simulink model "SVPWM"  (R2021a)
settings: Solver=VariableStepAuto  StartTime=0.0  StopTime=10.0  RelTol=1e-3
libraries: spsIGBTDiodeLib x6, spsSeriesRLCBranchLib x3, spsVoltageMeasurementLib x3, spsGroundLib x2, spsDCVoltageSourceLib x1, spsabctodq0Lib x1, spspowerguiLib x1
settings Model: Creator=User  LastModifiedBy=User

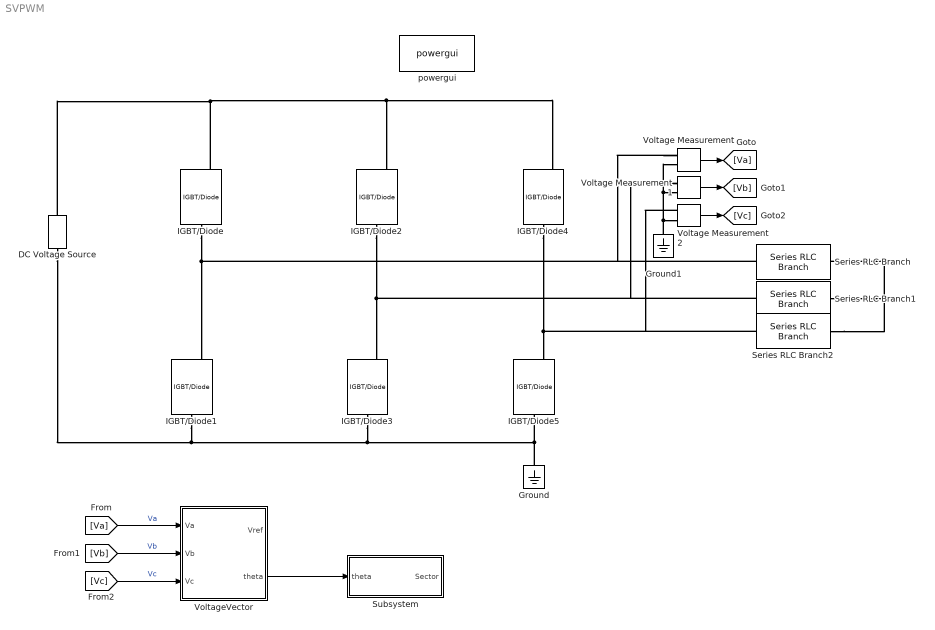
== system SVPWM ==
  DC Voltage Source : spsDCVoltageSourceLib/DC Voltage Source  Amplitude=100  Measurements=None
  Ground : spsGroundLib/Ground  LConnTagsString=a
  Ground1 : spsGroundLib/Ground  LConnTagsString=a
  IGBT/Diode{,1..5} (6 alike) : spsIGBTDiodeLib/IGBT//Diode  Ron=1e-3  Rs=1e5  Cs=inf  Measurements=off
  Series RLC Branch : spsSeriesRLCBranchLib/Series RLC Branch  LConnTagsString=__new0  RConnTagsString=__new0  BranchType=L  Resistance=1  Inductance=1e-3  SetiL0=off  InitialCurrent=0  Capacitance=1e-6  Setx0=off  InitialVoltage=0  Measurements=None
  Series RLC Branch1 : spsSeriesRLCBranchLib/Series RLC Branch  LConnTagsString=__new0  RConnTagsString=__new0  BranchType=L  Resistance=1  Inductance=1e-3  SetiL0=off  InitialCurrent=0  Capacitance=1e-6  Setx0=off  InitialVoltage=0  Measurements=None
  Series RLC Branch2 : spsSeriesRLCBranchLib/Series RLC Branch  LConnTagsString=__new0  RConnTagsString=__new0  BranchType=L  Resistance=1  Inductance=1e-3  SetiL0=off  InitialCurrent=0  Capacitance=1e-6  Setx0=off  InitialVoltage=0  Measurements=None
  Subsystem : Subsystem
  Voltage Measurement : spsVoltageMeasurementLib/Voltage Measurement  PhasorSimulation=off  OutputType=Complex  PSBequivalent=0
  Voltage Measurement1 : spsVoltageMeasurementLib/Voltage Measurement  PhasorSimulation=off  OutputType=Complex  PSBequivalent=0
  Voltage Measurement2 : spsVoltageMeasurementLib/Voltage Measurement  PhasorSimulation=off  OutputType=Complex  PSBequivalent=0
  VoltageVector : Subsystem
  powergui : spspowerguiLib/powergui  Priority=1  SimulationMode=Continuous  SampleTime=50e-6  frequency=60  Iterations=50  frequencyindice=60  Pbase=100e6  ErrMax=1e-4  UnitsV=kV  UnitsW=MW  buscounter=0  FunctionMessages=off  echomessages=off  EnableUseOfTLC=off  CurrentSourceSwitches=off  DisableSnubberDevices=off  DisableRonSwitches=off  DisableVfSwitches=off  DisplayEquations=off  AutomaticDiscreteSolvers=off  SolverType=Tustin/Backward Euler (TBE)  Interpol=off  ExternalGateDelay=off  methode=off  Ts=100  x0status=blocks  SPID=on  SwTol=0  HookPort=off  NonlinearTolerance=1e-4  nMaxIteration=100  ContinueOnMaxIteration=off  RestoreLinks=warning  ResistiveCurrentMeasurement=off  Frange=[0:2:500]  Ylog=off  Xlog=on  ShowGrid=off  save=off  variable=ZData  structure=0  ZoomFFT=off  StartTime=0.0  cycles=1  DisplayStyle=1  fundamental=60  FreqAxis=off  MaxFrequency=1000  frequencyindicesteady=1  RmsSteady=1  display=off
  wires:
  Voltage Measurement/1 -> [Va]
  Voltage Measurement1/1 -> [Vb]
  Voltage Measurement2/1 -> [Vc]
  [Va] -> VoltageVector/1(Va)  "Va"
  [Vb] -> VoltageVector/2(Vb)  "Vb"
  [Vc] -> VoltageVector/3(Vc)  "Vc"
  VoltageVector/2(theta) -> Subsystem/1(theta)
  connections:
  IGBT/Diode/LConn1 -- DC Voltage Source/RConn1 -- IGBT/Diode2/LConn1 -- IGBT/Diode4/LConn1
  IGBT/Diode2/RConn1 -- Voltage Measurement1/LConn1 -- Series RLC Branch1/LConn1 -- IGBT/Diode3/LConn1
  IGBT/Diode/RConn1 -- Voltage Measurement/LConn1 -- Series RLC Branch/LConn1 -- IGBT/Diode1/LConn1
  IGBT/Diode4/RConn1 -- Voltage Measurement2/LConn1 -- Series RLC Branch2/LConn1 -- IGBT/Diode5/LConn1
  IGBT/Diode1/RConn1 -- DC Voltage Source/LConn1 -- IGBT/Diode3/RConn1 -- Ground/LConn1 -- IGBT/Diode5/RConn1
  Series RLC Branch2/RConn1 -- Series RLC Branch1/RConn1 -- Series RLC Branch/RConn1
  Ground1/LConn1 -- Voltage Measurement1/LConn2 -- Voltage Measurement/LConn2 -- Voltage Measurement2/LConn2

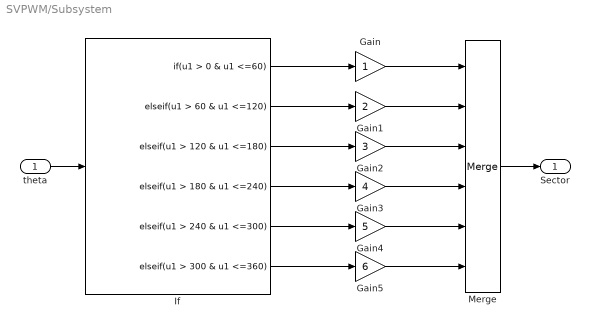
== system SVPWM/Subsystem ==
  theta : Inport
  Gain : Gain
  Gain1 : Gain  Gain=2
  Gain2 : Gain  Gain=3
  Gain3 : Gain  Gain=4
  Gain4 : Gain  Gain=5
  Gain5 : Gain  Gain=6
  If : If  IfExpression=u1 > 0 & u1 <=60  ElseIfExpressions=u1 > 60 & u1 <=120, u1 > 120 & u1 <=180, u1 > 180 & u1 <=240, u1 > 240 & u1 <=300, u1 > 300 & u1 <=360  ShowElse=off
  Merge : Merge  Inputs=6
  Sector : Outport
  wires:
  theta/1 -> If/1
  If/1 -> Gain/1
  If/2 -> Gain1/1
  If/3 -> Gain2/1
  If/4 -> Gain3/1
  If/5 -> Gain4/1
  If/6 -> Gain5/1
  Gain/1 -> Merge/1
  Gain1/1 -> Merge/2
  Gain2/1 -> Merge/3
  Gain3/1 -> Merge/4
  Gain4/1 -> Merge/5
  Gain5/1 -> Merge/6
  Merge/1 -> Sector/1

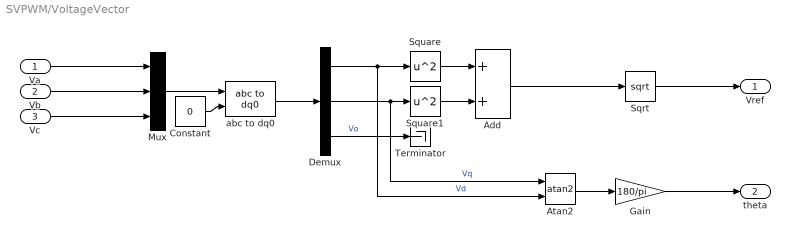
== system SVPWM/VoltageVector ==
  Va : Inport
  Vb : Inport  Port=2
  Vc : Inport  Port=3
  Add : Sum
  Atan2 : Trigonometry  Operator=atan2
  Constant : Constant  Value=0
  Demux : Demux  Outputs=3
  Gain : Gain  Gain=180/pi
  Mux : Mux  Inputs=3
      settings: DisplayOption=signals
  Sqrt : Sqrt  SaturateOnIntegerOverflow=on
  Square : Math  Operator=square  SaturateOnIntegerOverflow=on
  Square1 : Math  Operator=square  SaturateOnIntegerOverflow=on
  Terminator : Terminator
  abc to dq0 : spsabctodq0Lib/abc to dq0  Alignment=90 degrees behind phase A axis
  Vref : Outport
  theta : Outport  Port=2
  wires:
  Sqrt/1 -> Vref/1
  abc to dq0/1 -> Demux/1
  Constant/1 -> abc to dq0/2
  Square/1 -> Add/1
  Demux/1 -> Atan2/2, Square/1  "Vd"
  Square1/1 -> Add/2
  Mux/1 -> abc to dq0/1
  Demux/2 -> Atan2/1, Square1/1  "Vq"
  Vc/1 -> Mux/3
  Atan2/1 -> Gain/1
  Demux/3 -> Terminator/1  "Vo"
  Add/1 -> Sqrt/1
  Vb/1 -> Mux/2
  Gain/1 -> theta/1
  Va/1 -> Mux/1
